simulink model "flexible_joint_v11"  (R2023b)
settings: Solver=FixedStepAuto  StartTime=0.0  StopTime=50  FixedStep=0.001  RelTol=1e-3
libraries: slpidlib x2
settings Model: Creator=GreenTeam  LastModifiedBy=86188

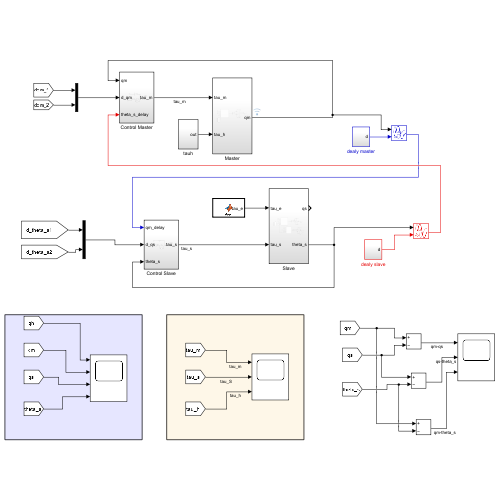
[thumbnail: Simulink's stored preview of the top-level diagram]
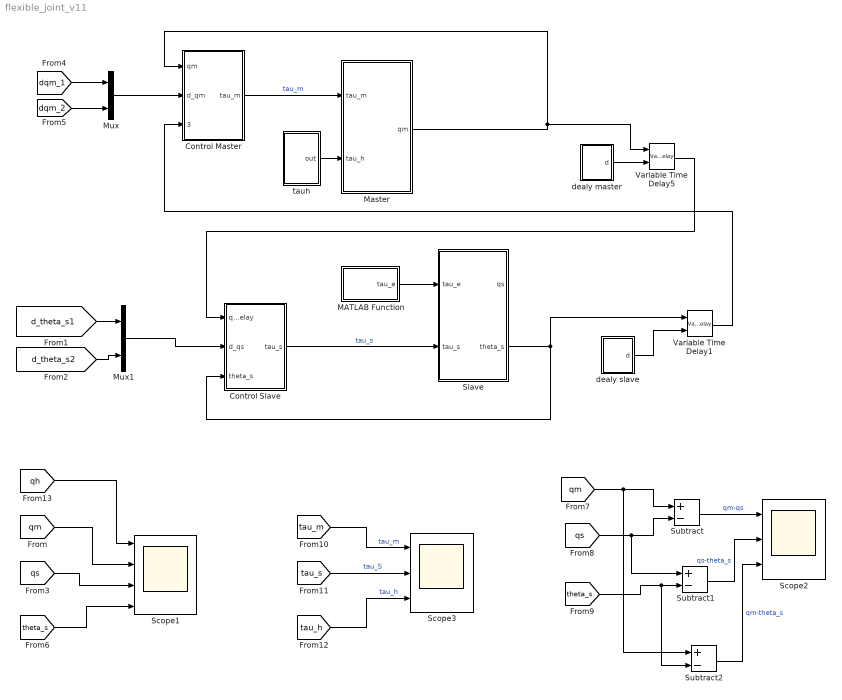
== system flexible_joint_v11 ==
  Control Master : Subsystem
  Control Slave : Subsystem
  MATLAB Function : MATLAB Function  TreatAsAtomicUnit=on
  Master : Subsystem
  Mux : Mux  Inputs=2
  Mux1 : Mux  Inputs=2
  Scope1 : Scope  NumInputPorts=4
  Scope2 : Scope  NumInputPorts=3
  Scope3 : Scope  NumInputPorts=3
  Slave : Subsystem
  Subtract : Sum  Inputs=+-
  Subtract1 : Sum  Inputs=+-
  Subtract2 : Sum  Inputs=+-
  Variable Time Delay1 : VariableTransportDelay  MaximumDelay=10  MaximumPoints=499712
  Variable Time Delay5 : VariableTransportDelay  MaximumDelay=10  MaximumPoints=499712
  dealy master : Subsystem
  dealy slave : Subsystem
  tauh : Subsystem
  wires:
  Variable Time Delay5/1 -> Control Slave/1(qm_delay)
  Variable Time Delay1/1 -> Control Master/3(theta_s_delay)
  dealy slave/1(d) -> Variable Time Delay1/2
  [qs] -> Subtract1/1, Subtract/2
  [d_theta_s2] -> Mux1/2
  [d_theta_s1] -> Mux1/1
  MATLAB Function/1(tau_e) -> Slave/1(tau_e)
  Subtract1/1 -> Scope2/2  "qs-theta_s"
  [dqm_2] -> Mux/2
  [qm] -> Scope1/2
  Master/1(qm) -> Variable Time Delay5/1, Control Master/1(qm)
  Subtract2/1 -> Scope2/3  "qm-theta_s"
  Slave/2(theta_s) -> Variable Time Delay1/1, Control Slave/3(theta_s)
  Mux/1 -> Control Master/2(d_qm)
  Mux1/1 -> Control Slave/2(d_qs)
  [theta_s] -> Scope1/4
  Control Master/1(tau_m) -> Master/1(tau_m)  "tau_m"
  [dqm_1] -> Mux/1
  Subtract/1 -> Scope2/1  "qm-qs"
  [theta_s] -> Subtract2/2, Subtract1/2
  [qm] -> Subtract2/1, Subtract/1
  [qs] -> Scope1/3
  dealy master/1(d) -> Variable Time Delay5/2
  Control Slave/1(tau_s) -> Slave/2(tau_s)  "tau_s"
  [tau_m] -> Scope3/1  "tau_m"
  [tau_h] -> Scope3/3  "tau_h"
  [tau_s] -> Scope3/2  "tau_S"
  [qh] -> Scope1/1
  tauh/1(out) -> Master/2(tau_h)

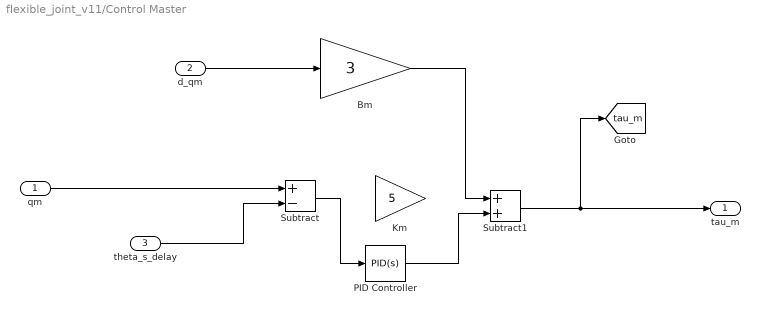
== system flexible_joint_v11/Control Master ==
  qm : Inport
  d_qm : Inport  Port=2
  theta_s_delay : Inport  Port=3
  Bm : Gain  Gain=3
  Km : Gain  Gain=5
  PID Controller : slpidlib/PID Controller  Controller=PID  Form=Parallel  TimeDomain=Continuous-time  UseExternalTs=off  SampleTime=-1  IntegratorMethod=Forward Euler  FilterMethod=Forward Euler  ControllerParametersSource=internal  P=30  I=0.5  UseKiTs=off  D=0.1  N=100  UseFilter=on  TunerSelectOption=Transfer Function Based (PID Tuner App)  InitialConditionSource=internal  InitialConditionForIntegrator=0  InitialConditionForFilter=0  DifferentiatorICPrevScaledInput=0  ExternalReset=none  TrackingMode=off  Kt=1  LimitOutput=off  SatLimitsSource=internal  UpperSaturationLimit=inf  LowerSaturationLimit=-inf  LinearizeAsGain=on  AntiWindupMode=none  Kb=1  LimitIntegrator=off  UpperIntegratorSaturationLimit=inf  LowerIntegratorSaturationLimit=-inf  POutMin=[]  POutMax=[]  IOutMin=[]  IOutMax=[]  DOutMin=[]  DOutMax=[]  NOutMin=[]  NOutMax=[]  SumOutMin=[]  SumOutMax=[]  SaturationOutMin=[]  SaturationOutMax=[]  PParamMin=[]  PParamMax=[]  IParamMin=[]  IParamMax=[]  DParamMin=[]  DParamMax=[]  NParamMin=[]  NParamMax=[]  KbParamMin=[]  KbParamMax=[]  KtParamMin=[]  KtParamMax=[]  KbOutMin=[]  KbOutMax=[]  KtOutMin=[]  KtOutMax=[]  IntegratorOutMin=[]  IntegratorOutMax=[]  FilterOutMin=[]  FilterOutMax=[]  SumI1OutMin=[]  SumI1OutMax=[]  SumI2OutMin=[]  SumI2OutMax=[]  SumI3OutMin=[]  SumI3OutMax=[]  SumI4OutMin=[]  SumI4OutMax=[]  SumDOutMin=[]  SumDOutMax=[]  DifferentiatorOutMin=[]  DifferentiatorOutMax=[]  FilterDiffOutCoefMin=[]  FilterDiffOutCoefMax=[]  ReciprocalOutMin=[]  ReciprocalOutMax=[]  SumDenOutMin=[]  SumDenOutMax=[]  SumNumOutMin=[]  SumNumOutMax=[]  DivideOutMin=[]  DivideOutMax=[]  UdiffTsProdOutMin=[]  UdiffTsProdOutMax=[]  NTsProdOutMin=[]  NTsProdOutMax=[]  UintegralTsProdOutMin=[]  UintegralTsProdOutMax=[]  UngainTsProdOutMin=[]  UngainTsProdOutMax=[]  ClampingZeroOutDataTypeStr=Inherit: Inherit via back propagation  ClampingZeroOutMin=[]  ClampingZeroOutMax=[]  FilterDenConstantOutDataTypeStr=Inherit: Inherit via back propagation  FilterDenConstantOutMin=[]  FilterDenConstantOutMax=[]  PCopyOutDataTypeStr=Inherit: Inherit via back propagation  PCopyOutMin=[]  PCopyOutMax=[]  NCopyOutDataTypeStr=Inherit: Inherit via back propagation  NCopyOutMin=[]  NCopyOutMax=[]  IntegratorContinuousStateAttributes=''  IntegratorStateMustResolveToSignalObject=off  IntegratorRTWStateStorageClass=Auto  FilterContinuousStateAttributes=''  FilterStateMustResolveToSignalObject=off  FilterRTWStateStorageClass=Auto  ParallelPVariant=InternalParameters  IdealPVariant=Disabled  IVariant=InternalParameters  DVariant=InternalParameters  IntegratorVariant=Continuous  SatVariant=Disabled  AWVariant=Passthrough  PCopyVariant=Disabled  TRVariant=Disabled  FdbkBlocksVariant=Forward  IdealPFdbkVariant=Disabled  SatFdbkVariant=Disabled  DerivativeFilterVariant=ContFilter  NVariant=InternalParameters  NCopyVariant=Disabled  FilterICVariant=InternalICsFilter  IntegratorICVariant=InternalICs  ExternalResetVariant=Disabled  TRSumVariant=Passthrough  SumFdbkVariant=Disabled  SumVariant=Sum_PID  TsampFilterVariant=InternalTs  TsampNgainVariant=Passthrough  TsampIntegralVariant=Disabled_SignalSpec  ExternalSaturationOutDataTypeStr=Inherit: Same as second input
  Subtract : Sum  Inputs=+-
  Subtract1 : Sum
  tau_m : Outport
  tag scope: tau_m=global
  wires:
  Bm/1 -> Subtract1/1
  Subtract/1 -> PID Controller/1
  Subtract1/1 -> [tau_m], tau_m/1
  PID Controller/1 -> Subtract1/2
  d_qm/1 -> Bm/1
  qm/1 -> Subtract/1
  theta_s_delay/1 -> Subtract/2

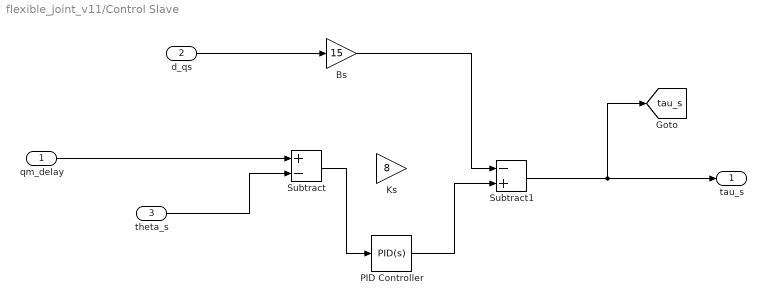
== system flexible_joint_v11/Control Slave ==
  qm_delay : Inport
  d_qs : Inport  Port=2
  theta_s : Inport  Port=3
  Bs : Gain  Gain=15
  Ks : Gain  Gain=8
  PID Controller : slpidlib/PID Controller  Controller=PID  Form=Parallel  TimeDomain=Continuous-time  UseExternalTs=off  SampleTime=-1  IntegratorMethod=Forward Euler  FilterMethod=Forward Euler  ControllerParametersSource=internal  P=20  I=1  UseKiTs=off  D=0.1  N=100  UseFilter=on  TunerSelectOption=Transfer Function Based (PID Tuner App)  InitialConditionSource=internal  InitialConditionForIntegrator=0  InitialConditionForFilter=0  DifferentiatorICPrevScaledInput=0  ExternalReset=none  TrackingMode=off  Kt=1  LimitOutput=off  SatLimitsSource=internal  UpperSaturationLimit=inf  LowerSaturationLimit=-inf  LinearizeAsGain=on  AntiWindupMode=none  Kb=1  LimitIntegrator=off  UpperIntegratorSaturationLimit=inf  LowerIntegratorSaturationLimit=-inf  POutMin=[]  POutMax=[]  IOutMin=[]  IOutMax=[]  DOutMin=[]  DOutMax=[]  NOutMin=[]  NOutMax=[]  SumOutMin=[]  SumOutMax=[]  SaturationOutMin=[]  SaturationOutMax=[]  PParamMin=[]  PParamMax=[]  IParamMin=[]  IParamMax=[]  DParamMin=[]  DParamMax=[]  NParamMin=[]  NParamMax=[]  KbParamMin=[]  KbParamMax=[]  KtParamMin=[]  KtParamMax=[]  KbOutMin=[]  KbOutMax=[]  KtOutMin=[]  KtOutMax=[]  IntegratorOutMin=[]  IntegratorOutMax=[]  FilterOutMin=[]  FilterOutMax=[]  SumI1OutMin=[]  SumI1OutMax=[]  SumI2OutMin=[]  SumI2OutMax=[]  SumI3OutMin=[]  SumI3OutMax=[]  SumI4OutMin=[]  SumI4OutMax=[]  SumDOutMin=[]  SumDOutMax=[]  DifferentiatorOutMin=[]  DifferentiatorOutMax=[]  FilterDiffOutCoefMin=[]  FilterDiffOutCoefMax=[]  ReciprocalOutMin=[]  ReciprocalOutMax=[]  SumDenOutMin=[]  SumDenOutMax=[]  SumNumOutMin=[]  SumNumOutMax=[]  DivideOutMin=[]  DivideOutMax=[]  UdiffTsProdOutMin=[]  UdiffTsProdOutMax=[]  NTsProdOutMin=[]  NTsProdOutMax=[]  UintegralTsProdOutMin=[]  UintegralTsProdOutMax=[]  UngainTsProdOutMin=[]  UngainTsProdOutMax=[]  ClampingZeroOutDataTypeStr=Inherit: Inherit via back propagation  ClampingZeroOutMin=[]  ClampingZeroOutMax=[]  FilterDenConstantOutDataTypeStr=Inherit: Inherit via back propagation  FilterDenConstantOutMin=[]  FilterDenConstantOutMax=[]  PCopyOutDataTypeStr=Inherit: Inherit via back propagation  PCopyOutMin=[]  PCopyOutMax=[]  NCopyOutDataTypeStr=Inherit: Inherit via back propagation  NCopyOutMin=[]  NCopyOutMax=[]  IntegratorContinuousStateAttributes=''  IntegratorStateMustResolveToSignalObject=off  IntegratorRTWStateStorageClass=Auto  FilterContinuousStateAttributes=''  FilterStateMustResolveToSignalObject=off  FilterRTWStateStorageClass=Auto  ParallelPVariant=InternalParameters  IdealPVariant=Disabled  IVariant=InternalParameters  DVariant=InternalParameters  IntegratorVariant=Continuous  SatVariant=Disabled  AWVariant=Passthrough  PCopyVariant=Disabled  TRVariant=Disabled  FdbkBlocksVariant=Forward  IdealPFdbkVariant=Disabled  SatFdbkVariant=Disabled  DerivativeFilterVariant=ContFilter  NVariant=InternalParameters  NCopyVariant=Disabled  FilterICVariant=InternalICsFilter  IntegratorICVariant=InternalICs  ExternalResetVariant=Disabled  TRSumVariant=Passthrough  SumFdbkVariant=Disabled  SumVariant=Sum_PID  TsampFilterVariant=InternalTs  TsampNgainVariant=Passthrough  TsampIntegralVariant=Disabled_SignalSpec  ExternalSaturationOutDataTypeStr=Inherit: Same as second input
  Subtract : Sum  Inputs=+-
  Subtract1 : Sum  Inputs=-+
  tau_s : Outport
  tag scope: tau_s=global
  wires:
  theta_s/1 -> Subtract/2
  qm_delay/1 -> Subtract/1
  d_qs/1 -> Bs/1
  PID Controller/1 -> Subtract1/2
  Subtract1/1 -> [tau_s], tau_s/1
  Subtract/1 -> PID Controller/1
  Bs/1 -> Subtract1/1

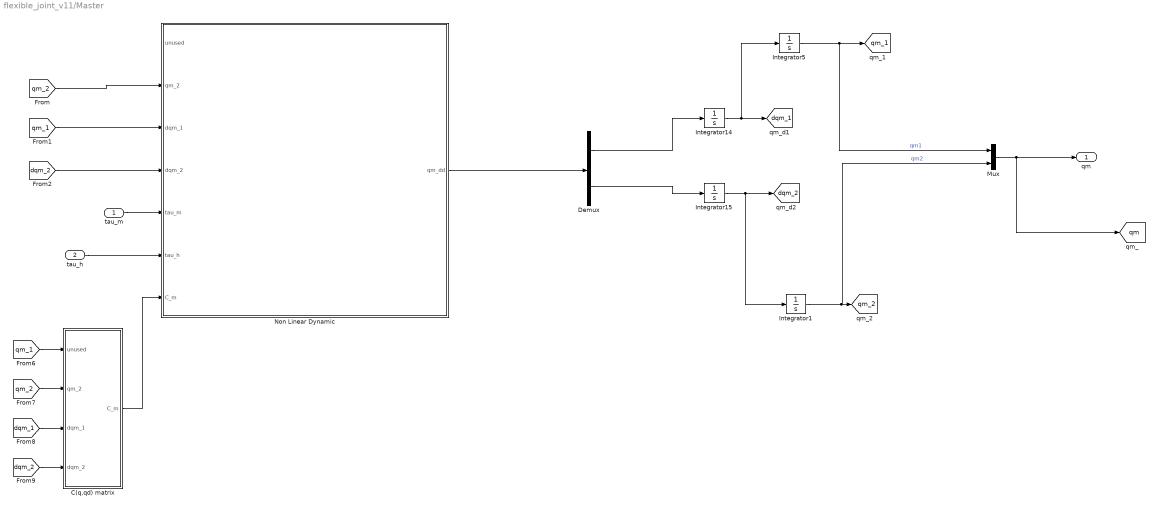
== system flexible_joint_v11/Master ==
  tau_m : Inport
  tau_h : Inport  Port=2
  C(q,qd) matrix : MATLAB Function  TreatAsAtomicUnit=on
  Demux : Demux  Outputs=2
  Integrator1 : Integrator  InitialCondition=pi/8
  Integrator14 : Integrator
  Integrator15 : Integrator
  Integrator5 : Integrator  InitialCondition=-pi/8
  Mux : Mux  Inputs=2
  Non Linear Dynamic : MATLAB Function  TreatAsAtomicUnit=on
  qm : Outport  VectorParamsAs1DForOutWhenUnconnected=off
  tag scope: dqm_1=global, dqm_2=global, qm=global, qm_1=global, qm_2=global
  wires:
  Integrator5/1 -> Mux/1, [qm_1]  "qm1"
  Demux/1 -> Integrator14/1
  Non Linear Dynamic/1(qm_dd) -> Demux/1
  Integrator1/1 -> Mux/2, [qm_2]  "qm2"
  tau_m/1 -> Non Linear Dynamic/5(tau_m)
  Integrator14/1 -> Integrator5/1, [dqm_1]
  Integrator15/1 -> Integrator1/1, [dqm_2]
  Demux/2 -> Integrator15/1
  C(q,qd) matrix/1(C_m) -> Non Linear Dynamic/7(C_m)
  [qm_2] -> Non Linear Dynamic/2(qm_2)
  [dqm_2] -> Non Linear Dynamic/4(dqm_2)
  [qm_1] -> Non Linear Dynamic/3(dqm_1)
  [dqm_1] -> C(q,qd) matrix/3(dqm_1)
  [qm_1] -> C(q,qd) matrix/1(unused)
  [dqm_2] -> C(q,qd) matrix/4(dqm_2)
  [qm_2] -> C(q,qd) matrix/2(qm_2)
  Mux/1 -> [qm], qm/1
  tau_h/1 -> Non Linear Dynamic/6(tau_h)

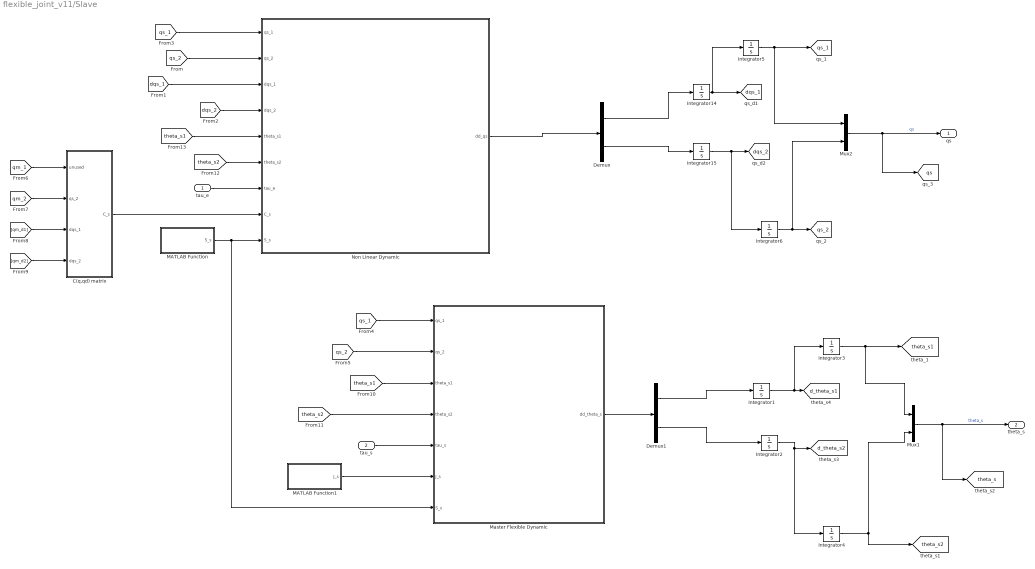
== system flexible_joint_v11/Slave ==
  tau_e : Inport
  tau_s : Inport  Port=2
  C(q,qd) matrix : MATLAB Function  TreatAsAtomicUnit=on
  Demux : Demux  Outputs=2
  Demux1 : Demux  Outputs=2
  Integrator{1..2,14..15} (4 alike) : Integrator
  Integrator3 : Integrator  InitialCondition=pi/5
  Integrator4 : Integrator  InitialCondition=-1/2*pi
  Integrator5 : Integrator  InitialCondition=1/5*pi
  Integrator6 : Integrator  InitialCondition=-1/2*pi
  MATLAB Function : MATLAB Function  TreatAsAtomicUnit=on
  MATLAB Function1 : MATLAB Function  TreatAsAtomicUnit=on
  Master Flexible Dynamic : MATLAB Function  TreatAsAtomicUnit=on
  Mux1 : Mux  Inputs=2
  Mux2 : Mux  Inputs=2
  Non Linear Dynamic : MATLAB Function  TreatAsAtomicUnit=on
  qs : Outport
  theta_s : Outport  Port=2
  tag scope: d_theta_s1=global, d_theta_s2=global, dqs_1=global, dqs_2=global, qs=global, qs_1=global, qs_2=global, theta_s1=global, theta_s2=global, theta_s=global
  wires:
  [qm_2] -> C(q,qd) matrix/2(qs_2)
  [qm_d2] -> C(q,qd) matrix/4(dqs_2)
  [qm_1] -> C(q,qd) matrix/1(unused)
  [qm_d1] -> C(q,qd) matrix/3(dqs_1)
  [dqs_1] -> Non Linear Dynamic/3(dqs_1)
  [dqs_2] -> Non Linear Dynamic/4(dqs_2)
  [qs_2] -> Non Linear Dynamic/2(qs_2)
  Demux/2 -> Integrator15/1
  Integrator15/1 -> Integrator6/1, [dqs_2]
  Integrator14/1 -> [dqs_1], Integrator5/1
  Integrator6/1 -> Mux2/2, [qs_2]
  Non Linear Dynamic/1(dd_qs) -> Demux/1
  Demux/1 -> Integrator14/1
  Mux2/1 -> [qs], qs/1  "qs"
  Integrator5/1 -> Mux2/1, [qs_1]
  C(q,qd) matrix/1(C_s) -> Non Linear Dynamic/8(C_s)
  MATLAB Function/1(S_s) -> Non Linear Dynamic/9(S_s), Master Flexible Dynamic/7(S_s)
  [qs_1] -> Non Linear Dynamic/1(qs_1)
  MATLAB Function1/1(J_s) -> Master Flexible Dynamic/6(J_s)
  Integrator3/1 -> Mux1/1, [theta_s1]
  Integrator1/1 -> Integrator3/1, [d_theta_s1]
  Demux1/1 -> Integrator1/1
  Master Flexible Dynamic/1(dd_theta_s) -> Demux1/1
  Integrator4/1 -> [theta_s2], Mux1/2
  Integrator2/1 -> Integrator4/1, [d_theta_s2]
  Mux1/1 -> [theta_s], theta_s/1  "theta_s"
  Demux1/2 -> Integrator2/1
  [qs_1] -> Master Flexible Dynamic/1(qs_1)
  [qs_2] -> Master Flexible Dynamic/2(qs_2)
  [theta_s1] -> Master Flexible Dynamic/3(theta_s1)
  [theta_s2] -> Master Flexible Dynamic/4(theta_s2)
  [theta_s2] -> Non Linear Dynamic/6(theta_s2)
  [theta_s1] -> Non Linear Dynamic/5(theta_s1)
  tau_e/1 -> Non Linear Dynamic/7(tau_e)
  tau_s/1 -> Master Flexible Dynamic/5(tau_s)

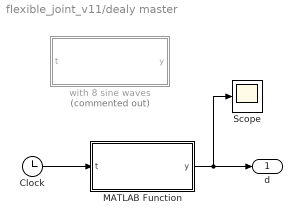
== system flexible_joint_v11/dealy master ==
  Clock : Clock
  MATLAB Function : MATLAB Function  TreatAsAtomicUnit=on
  Scope : Scope
  with 8 sine waves : MATLAB Function  Commented=on  TreatAsAtomicUnit=on
  d : Outport
  wires:
  MATLAB Function/1(y) -> Scope/1, d/1
  Clock/1 -> MATLAB Function/1(t)

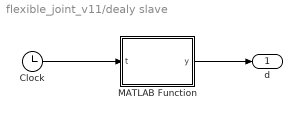
== system flexible_joint_v11/dealy slave ==
  Clock : Clock
  MATLAB Function : MATLAB Function  TreatAsAtomicUnit=on
  d : Outport
  wires:
  Clock/1 -> MATLAB Function/1(t)
  MATLAB Function/1(y) -> d/1

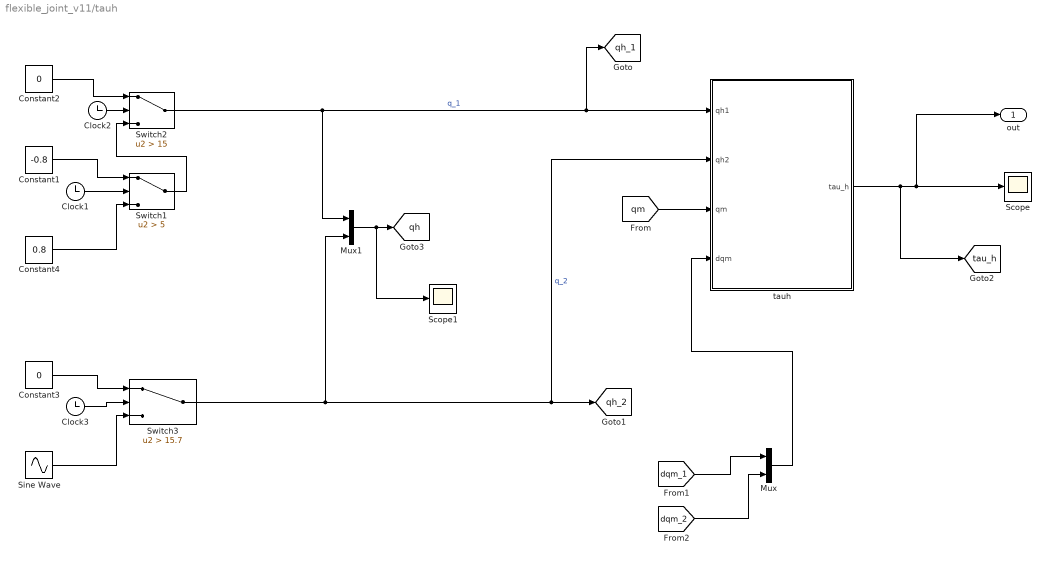
== system flexible_joint_v11/tauh ==
  Clock1 : Clock
  Clock2 : Clock
  Clock3 : Clock
  Constant1 : Constant  Value=-0.8
  Constant2 : Constant  Value=0
  Constant3 : Constant  Value=0
  Constant4 : Constant  Value=0.8
  Mux : Mux  Inputs=2
  Mux1 : Mux  Inputs=2
  Scope : Scope
  Scope1 : Scope
  Sine Wave : Sin  Amplitude=1.5  Frequency=0.2  SampleTime=0
  Switch1 : Switch  Criteria=u2 > Threshold  Threshold=5  SaturateOnIntegerOverflow=off  InputSameDT=off
  Switch2 : Switch  Criteria=u2 > Threshold  Threshold=15  SaturateOnIntegerOverflow=off  InputSameDT=off
  Switch3 : Switch  Criteria=u2 > Threshold  Threshold=15.7  SaturateOnIntegerOverflow=off  InputSameDT=off
  tauh : MATLAB Function  TreatAsAtomicUnit=on
  out : Outport
  tag scope: qh=global, qh_1=global, qh_2=global, tau_h=global
  wires:
  tauh/1(tau_h) -> [tau_h], out/1, Scope/1
  Switch3/1 -> Mux1/2, tauh/2(qh2), [qh_2]  "q_2"
  Switch2/1 -> Mux1/1, [qh_1], tauh/1(qh1)  "q_1"
  Sine Wave/1 -> Switch3/3
  Clock3/1 -> Switch3/2
  Constant3/1 -> Switch3/1
  Constant1/1 -> Switch1/1
  Constant2/1 -> Switch2/1
  Clock2/1 -> Switch2/2
  Switch1/1 -> Switch2/3
  Clock1/1 -> Switch1/2
  Constant4/1 -> Switch1/3
  [dqm_1] -> Mux/1
  [dqm_2] -> Mux/2
  Mux/1 -> tauh/4(dqm)
  [qm] -> tauh/3(qm)
  Mux1/1 -> Scope1/1, [qh]

== matlab function flexible_joint_v11/dealy slave/MATLAB Function ==
  data: t input; y output
function y = reconstructed_signal(t)
    % Given data
    DC_offset = 0.9613462407597305;
    sine_amplitudes = [-0.02000659, -0.02349457, 0.00067474, 0.00159032, 0.00129016, -0.00135477, -0.00022001, 0.00097632, 0.00021585, 0.00014519, -0.00020833, -0.00056968, -0.00031181, 0.00016964, 0.0003376, -0.00022124];
    cosine_amplitudes = [-0.02556397, 0.00393168, -0.0052079, 0.00220769, 0.00300956, 0.00160663, -0.00018929, -0.00031848, -0.00019025, -0.00022222, -0.00010147, 0.00019351, -0.00030343, 0.0001225, 0.00015061, 0.00039704];
    frequencies = [0.24299065416927243, 0.48598130833854486, 0.7289719625078173, 0.9719626166770897, 1.2149532708463622, 1.4579439250156345, 1.7009345791849069, 1.9439252333541794, 2.186915887523452, 2.4299065416927244, 2.6728971958619967, 2.915887850031269, 3.1588785042005414, 3.4018691583698137, 3.6448598125390865, 3.887850466708359];
    
    % Number of terms
    N = length(sine_amplitudes);
    
    % Initialize the signal
    y = DC_offset * ones(size(t));
    
    % Add sine and cosine terms
    for k = 1:N
        y = y + sine_amplitudes(k) * sin(2 * pi * frequencies(k) * t) + cosine_amplitudes(k) * cos(2 * pi * frequencies(k) * t);
    end
end

== matlab function flexible_joint_v11/dealy master/with 8 sine waves ==
  data: t input; y output
function y = reconstructed_signal(t)
    % Given data
    DC_offset = 0.9613888244716796;
    sine_amplitudes = [-0.02002779, -0.02351674, 0.00074362, 0.00154452, 0.0013555, -0.00135695, -0.00015931, 0.00089033];
    cosine_amplitudes = [-0.02562599, 0.00393932, -0.00523797, 0.0022634, 0.00295895, 0.00158273, -0.00018019, -0.0003756];
    frequencies = [0.24299065416927243, 0.48598130833854486, 0.7289719625078173, 0.9719626166770897, 1.2149532708463622, 1.4579439250156345, 1.7009345791849069, 1.9439252333541794];
    
    % Number of terms
    N = length(sine_amplitudes);
    
    % Initialize the signal
    y = DC_offset * ones(size(t));
    
    % Add sine and cosine terms
    for k = 1:N
        y = y + sine_amplitudes(k) * sin(2 * pi * frequencies(k) * t) + cosine_amplitudes(k) * cos(2 * pi * frequencies(k) * t);
    end
end

== matlab function flexible_joint_v11/tauh/tauh ==
  data: qh1 input; qh2 input; qm input; tau_h output; dqm input
function tau_h = spring_damper(qh1,qh2,qm,dqm)

Kh=10;
Dh=2;

qh=[qh1;qh2];
tau_h=Kh*(qh-qm)-Dh*dqm;


end

== matlab function flexible_joint_v11/Master/C(q,qd) matrix ==
  data: unused input; qm_2 input; dqm_1 input; C_m output; dqm_2 input
function C_m = fcn(~,qm_2,dqm_1,dqm_2)

% Phyiscal Parameters
Lm1 = 0.38;                                          %Master_first_link_length
Lm2 = 0.38;                                          %Master_second_link_length
mm1 = 3.5;                                           %Master_first_link_mass
mm2 = 0.5;                                           %Master_second_link_mass

betha_m=Lm1*Lm2*mm2;

C_m_11 = -2*betha_m*sin(qm_2)*dqm_2;
C_m_12 = -betha_m*sin(qm_2)*dqm_2;
C_m_21 =  betha_m*sin(qm_2)*dqm_1;
C_m_22 =  0;
C_m = [C_m_11 C_m_12; C_m_21 C_m_22];
end

== matlab function flexible_joint_v11/dealy master/MATLAB Function ==
  data: t input; y output
function y = reconstructed_signal(t)
    % Given data
    DC_offset = 0.9613462407597305;
    sine_amplitudes = [-0.02000659, -0.02349457, 0.00067474, 0.00159032, 0.00129016, -0.00135477, -0.00022001, 0.00097632, 0.00021585, 0.00014519, -0.00020833, -0.00056968, -0.00031181, 0.00016964, 0.0003376, -0.00022124];
    cosine_amplitudes = [-0.02556397, 0.00393168, -0.0052079, 0.00220769, 0.00300956, 0.00160663, -0.00018929, -0.00031848, -0.00019025, -0.00022222, -0.00010147, 0.00019351, -0.00030343, 0.0001225, 0.00015061, 0.00039704];
    frequencies = [0.24299065416927243, 0.48598130833854486, 0.7289719625078173, 0.9719626166770897, 1.2149532708463622, 1.4579439250156345, 1.7009345791849069, 1.9439252333541794, 2.186915887523452, 2.4299065416927244, 2.6728971958619967, 2.915887850031269, 3.1588785042005414, 3.4018691583698137, 3.6448598125390865, 3.887850466708359];
    
    % Number of terms
    N = length(sine_amplitudes);
    
    % Initialize the signal
    y = DC_offset * ones(size(t));
    
    % Add sine and cosine terms
    for k = 1:N
        y = y + sine_amplitudes(k) * sin(2 * pi * frequencies(k) * t) + cosine_amplitudes(k) * cos(2 * pi * frequencies(k) * t);
    end
end

== matlab function flexible_joint_v11/Master/Non Linear Dynamic ==
  data: unused input; qm_2 input; dqm_1 input; dqm_2 input; tau_m input; tau_h input; qm_dd output; C_m input
function qm_dd =fcn(~,qm_2,dqm_1,dqm_2,tau_m,tau_h,C_m)

% Phyiscal Parameters
Lm1 = 0.38;                                          %Master_first_link_length
Lm2 = 0.38;                                          %Master_second_link_length
mm1 = 3.5;                                           %Master_first_link_mass
mm2 = 0.5;                                           %Master_second_link_mass

dqm=[dqm_1;dqm_2];
alpha_m=(Lm2^2)*mm2+(Lm1^2)*(mm1+mm2);
betha_m=Lm1*Lm2*mm2;
delta_m=(Lm2^2)*mm2;

M_m_11= alpha_m + 2*betha_m*cos(qm_2);  
M_m_12= delta_m + betha_m * cos(qm_2);
M_m_21= M_m_12;
M_m_22= delta_m;
M_m = [M_m_11 M_m_12; M_m_21 M_m_22];
qm_dd = inv(M_m)*( -tau_m -(C_m * dqm ) + tau_h );
end

== matlab function flexible_joint_v11/Slave/C(q,qd) matrix ==
  data: unused input; qs_2 input; dqs_1 input; C_s output; dqs_2 input
function C_s = fcn(~,qs_2,dqs_1,dqs_2)

% Phyiscal Parameters
Ls1 = 0.3265;          % Link 1 length (m)
Ls2 = 0.3265;          % Link 2 length (m)

ms1 = 0.5362;          % Link 1 mass (kg)
ms2 = 0.5362;          % Link 2 mass (kg)

betha_s=Ls1*Ls2*ms2;

C_s_11 = -2*betha_s*sin(qs_2)*dqs_2;
C_s_12 = -betha_s*sin(qs_2)*dqs_2;
C_s_21 =  betha_s*sin(qs_2)*dqs_1;
C_s_22 =  0;
C_s= [C_s_11 C_s_12; C_s_21 C_s_22];
end

== matlab function flexible_joint_v11/Slave/MATLAB Function ==
  data: S_s output
function S_s = Stifness_Matrix()
    % This function creates a 2x2 identity matrix scaled by 500

    % Create a 2x2 identity matrix
    I = eye(2);
    
    % Scale the identity matrix by 500
    S_s = 500 * I;
end

== matlab function flexible_joint_v11/Slave/Master Flexible Dynamic ==
  data: qs_1 input; qs_2 input; theta_s1 input; dd_theta_s output; theta_s2 input; tau_s input; J_s input; S_s input
function dd_theta_s = Flex_Body_Slave(qs_1,qs_2,theta_s1,theta_s2,tau_s,J_s,S_s)

qs=[qs_1;qs_2];
theta_s=[theta_s1;theta_s2];


dd_theta_s = inv(J_s)*(tau_s - S_s*(theta_s-qs));

end

== matlab function flexible_joint_v11/Slave/MATLAB Function1 ==
  data: J_s output
function J_s = Inertia_Matrix()

    % Create a 2x2 identity matrix
    I = eye(2);
    % Scale the identity matrix by 500
    J_s = 0.2 * I;
end

== matlab function flexible_joint_v11/MATLAB Function ==
  data: tau_e output
function tau_e = fcn()

tau_e=[0;0];

== matlab function flexible_joint_v11/Slave/Non Linear Dynamic ==
  data: qs_1 input; qs_2 input; dqs_1 input; dqs_2 input; theta_s1 input; theta_s2 input; dd_qs output; tau_e input; C_s input; S_s input
function dd_qs =Rigid_Body_Slave(qs_1,qs_2,dqs_1,dqs_2,theta_s1,theta_s2,tau_e,C_s,S_s)

%% Physical Parameters (According to the experimental platform)

Ls1 = 0.3265;          % Link 1 length (m)
Ls2 = 0.3265;          % Link 2 length (m)

ms1 = 0.5362;          % Link 1 mass (kg)
ms2 = 0.5362;          % Link 2 mass (kg)

%% State Variables

qs      = [qs_1;qs_2];
theta_s = [theta_s1;theta_s2];
dqs     = [dqs_1;dqs_2];

%% Dynamic Parameters

alpha_s = (Ls2^2)*ms2 + (Ls1^2)*(ms1+ms2);
beta_s  = Ls1*Ls2*ms2;
delta_s = (Ls2^2)*ms2;

%% Inertia Matrix

M_s = [ alpha_s + 2*beta_s*cos(qs_2),  delta_s + beta_s*cos(qs_2);
        delta_s + beta_s*cos(qs_2),    delta_s ];

%% Dynamics
dd_qs= inv(M_s)*(- tau_e  - (C_s * dqs ) - (S_s*(qs-theta_s)));
end
